simulink model "sim_model"  (R2015b)
settings: Solver=FixedStepDiscrete  SolverMode=SingleTasking  StartTime=0.0  StopTime=sim_len  FixedStep=1  RelTol=1e-3
values from neighbouring files (symbols this model uses):
  N_sub = 16    [channelizer_params.m]    (also in channelizer_params_256.m = 256; channelizer_params_512.m = 512)
undefined symbols (not defined in the file or in its folder): modulator_reg_1_address, modulator_reg_1_default, modulator_reg_1_num_bits
libraries: xbsIndex_r4 x150
(part 1 of 2)
settings Model: Creator=randy  LastModifiedBy=randy

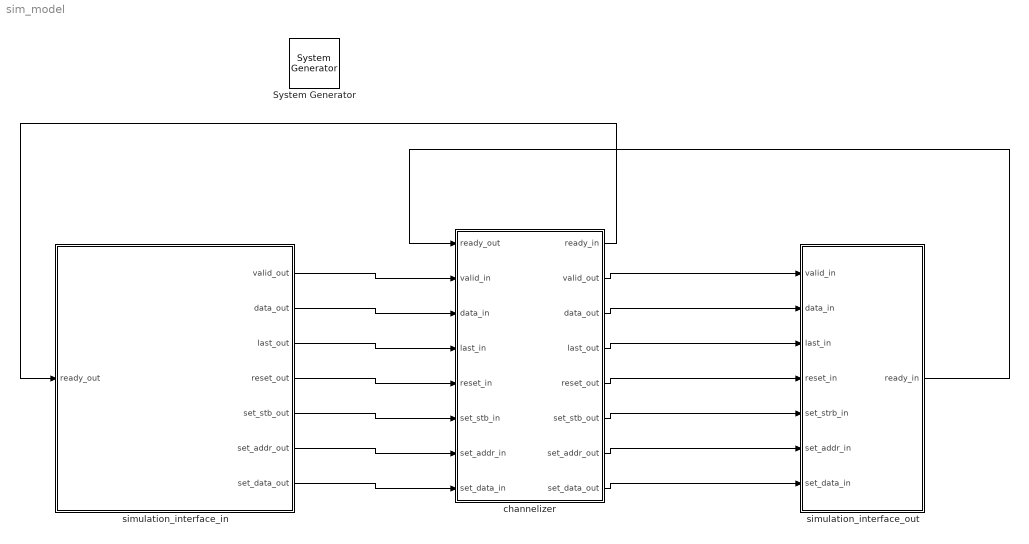
== system sim_model ==
  " System Generator" : xbsIndex_r4/ System Generator  Tag=genX  xilinxfamily=kintex7  part=xc7k325t  speed=-3  package=fbg676  synthesis_tool=Vivado  clock_wrapper=Clock Enables  directory=./netlist  proj_type=Vivado  Synth_file=Vivado Synthesis Defaults  Impl_file=Vivado Implementation Defaults  testbench=off  simulink_period=1  sysclk_period=10  dcm_input_clock_period=10  incr_netlist=off  trim_vbits=Everywhere in SubSystem  dbl_ovrd=According to Block Masks  core_generation=According to Block Masks  run_coregen=off  deprecated_control=off  eval_field=0  block_type=sysgen
  channelizer : Subsystem
  simulation_interface_in : Subsystem
  simulation_interface_out : Subsystem
  wires:
  channelizer/1(ready_in) -> simulation_interface_in/1(ready_out)
  channelizer/2(valid_out) -> simulation_interface_out/1(valid_in)
  channelizer/3(data_out) -> simulation_interface_out/2(data_in)
  channelizer/4(last_out) -> simulation_interface_out/3(last_in)
  simulation_interface_out/1(ready_in) -> channelizer/1(ready_out)
  channelizer/5(reset_out) -> simulation_interface_out/4(reset_in)
  channelizer/6(set_stb_out) -> simulation_interface_out/5(set_strb_in)
  channelizer/7(set_addr_out) -> simulation_interface_out/6(set_addr_in)
  channelizer/8(set_data_out) -> simulation_interface_out/7(set_data_in)
  simulation_interface_in/1(valid_out) -> channelizer/2(valid_in)
  simulation_interface_in/2(data_out) -> channelizer/3(data_in)
  simulation_interface_in/3(last_out) -> channelizer/4(last_in)
  simulation_interface_in/4(reset_out) -> channelizer/5(reset_in)
  simulation_interface_in/5(set_stb_out) -> channelizer/6(set_stb_in)
  simulation_interface_in/6(set_addr_out) -> channelizer/7(set_addr_in)
  simulation_interface_in/7(set_data_out) -> channelizer/8(set_data_in)

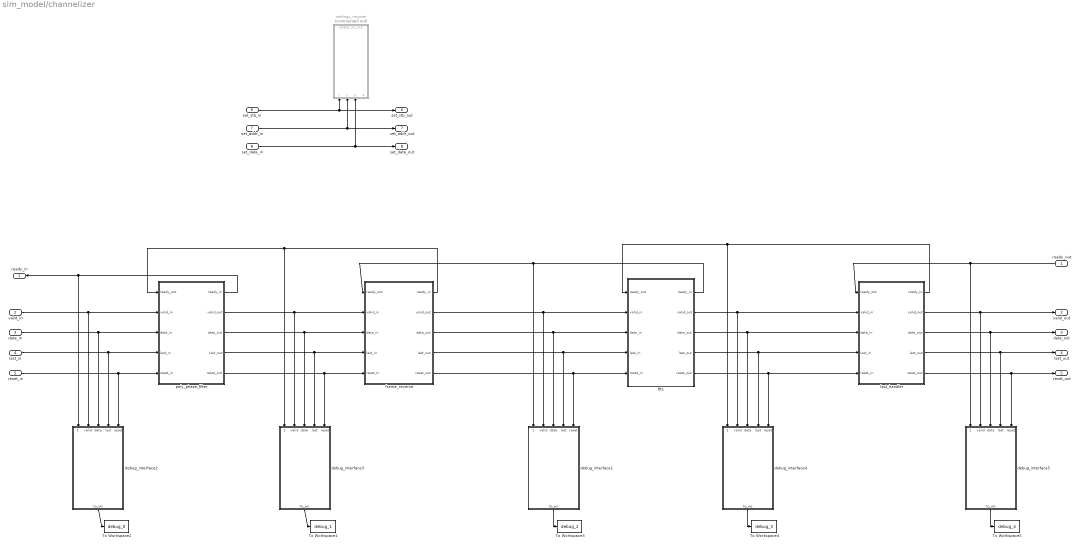
== system sim_model/channelizer ==
  ready_out : Inport
  valid_in : Inport  Port=2
  data_in : Inport  Port=3
  last_in : Inport  Port=4
  reset_in : Inport  Port=5
  set_stb_in : Inport  Port=6
  set_addr_in : Inport  Port=7
  set_data_in : Inport  Port=8
  To Workspace1 : ToWorkspace  VariableName=debug_1  SaveFormat=Timeseries  SampleTime=-1
  To Workspace2 : ToWorkspace  VariableName=debug_0  SaveFormat=Timeseries  SampleTime=-1
  To Workspace3 : ToWorkspace  VariableName=debug_2  SaveFormat=Timeseries  SampleTime=-1
  To Workspace4 : ToWorkspace  VariableName=debug_3  SaveFormat=Timeseries  SampleTime=-1
  To Workspace5 : ToWorkspace  VariableName=debug_4  SaveFormat=Timeseries  SampleTime=-1
  debug_interface1 : Subsystem
  debug_interface2 : Subsystem
  debug_interface3 : Subsystem
  debug_interface4 : Subsystem
  debug_interface5 : Subsystem
  fft1 : Subsystem
  frame_reverse : Subsystem
  last_handler : Subsystem
  poly_phase_filter : Subsystem
  settings_register : Subsystem  Commented=on
  ready_in : Outport
  valid_out : Outport  Port=2
  data_out : Outport  Port=3
  last_out : Outport  Port=4
  reset_out : Outport  Port=5
  set_stb_out : Outport  Port=6
  set_addr_out : Outport  Port=7
  set_data_out : Outport  Port=8
  wires:
  set_stb_in/1 -> settings_register/1(set_stb), set_stb_out/1
  set_addr_in/1 -> settings_register/2(set_addr), set_addr_out/1
  set_data_in/1 -> settings_register/3(set_data), set_data_out/1
  debug_interface2/1(to_ws) -> To Workspace2/1
  debug_interface3/1(to_ws) -> To Workspace1/1
  debug_interface1/1(to_ws) -> To Workspace3/1
  debug_interface4/1(to_ws) -> To Workspace4/1
  poly_phase_filter/1(ready_in) -> debug_interface2/1(ready), ready_in/1
  data_in/1 -> poly_phase_filter/3(data_in), debug_interface2/3(data)
  valid_in/1 -> poly_phase_filter/2(valid_in), debug_interface2/2(valid)
  last_in/1 -> poly_phase_filter/4(last_in), debug_interface2/4(last)
  reset_in/1 -> poly_phase_filter/5(reset_in), debug_interface2/5(reset)
  poly_phase_filter/2(valid_out) -> frame_reverse/2(valid_in), debug_interface3/2(valid)
  poly_phase_filter/3(data_out) -> frame_reverse/3(data_in), debug_interface3/3(data)
  poly_phase_filter/4(last_out) -> frame_reverse/4(last_in), debug_interface3/4(last)
  poly_phase_filter/5(reset_out) -> debug_interface3/5(reset), frame_reverse/5(reset_in)
  frame_reverse/2(valid_out) -> fft1/2(valid_in), debug_interface1/2(valid)
  frame_reverse/4(last_out) -> fft1/4(last_in), debug_interface1/4(last)
  frame_reverse/5(reset_out) -> fft1/5(reset_in), debug_interface1/5(reset)
  fft1/1(ready_in) -> frame_reverse/1(ready_out), debug_interface1/1(ready)
  frame_reverse/3(data_out) -> fft1/3(data_in), debug_interface1/3(data)
  frame_reverse/1(ready_in) -> poly_phase_filter/1(ready_out), debug_interface3/1(ready)
  last_handler/5(reset_out) -> reset_out/1, debug_interface5/5(reset)
  last_handler/4(last_out) -> last_out/1, debug_interface5/4(last)
  last_handler/3(data_out) -> data_out/1, debug_interface5/3(data)
  fft1/2(valid_out) -> debug_interface4/2(valid), last_handler/2(valid_in)
  fft1/3(data_out) -> debug_interface4/3(data), last_handler/3(data_in)
  fft1/4(last_out) -> debug_interface4/4(last), last_handler/4(last_in)
  fft1/5(reset_out) -> debug_interface4/5(reset), last_handler/5(reset_in)
  last_handler/2(valid_out) -> debug_interface5/2(valid), valid_out/1
  ready_out/1 -> debug_interface5/1(ready), last_handler/1(ready_out)
  last_handler/1(ready_in) -> debug_interface4/1(ready), fft1/1(ready_out)
  debug_interface5/1(to_ws) -> To Workspace5/1

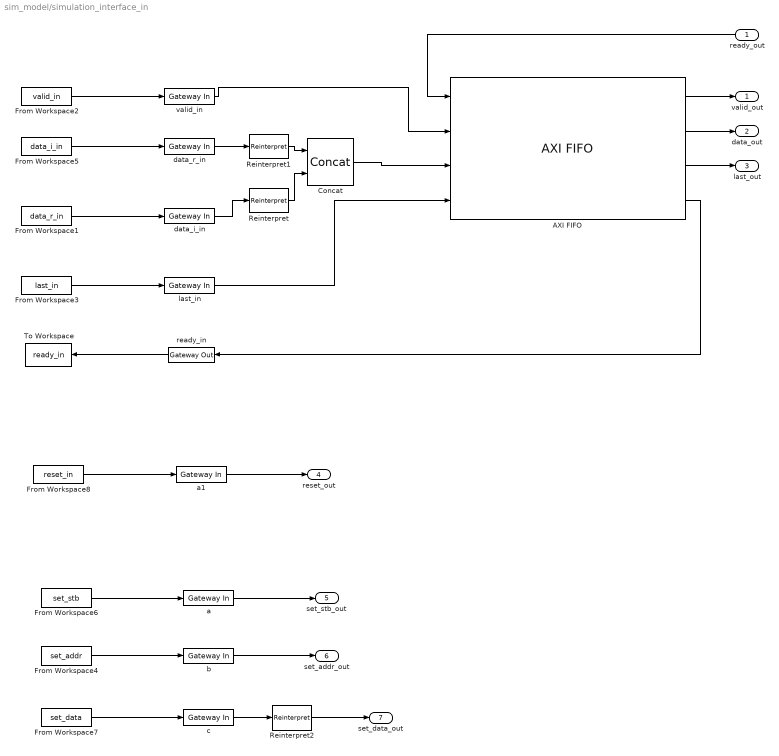
== system sim_model/simulation_interface_in ==
  ready_out : Inport
  AXI FIFO : xbsIndex_r4/AXI FIFO  input_depth_axis=16K  actual_fifo_depth_label=16386  enable_tdata=on  enable_tdest=off  enable_tstrb=off  enable_tready=on  enable_tid=off  enable_tuser=off  enable_tkeep=off  enable_tlast=on  has_aresetn=off  enable_data_counts_axis=off  fifo_implementation_type_axis=Common Clock Block RAM  trim_axipin_name=on  programmable_full_type_axis=Full  full_threshold_assert_value_axis=0  programmable_empty_type_axis=Empty  empty_threshold_assert_value_axis=1022  underflow_flag_axi=0  underflow_sense_axi=Active High  overflow_flag_axi=0  overflow_sense_axi=Active High  block_type=axi_fifo
  Concat : xbsIndex_r4/Concat  num_inputs=2  dbl_ovrd=off  block_type=concat
  From Workspace1 : FromWorkspace  VariableName=data_r_in  SampleTime=0
  From Workspace2 : FromWorkspace  VariableName=valid_in  SampleTime=0
  From Workspace3 : FromWorkspace  VariableName=last_in  SampleTime=0
  From Workspace4 : FromWorkspace  VariableName=set_addr  SampleTime=0
  From Workspace5 : FromWorkspace  VariableName=data_i_in  SampleTime=0
  From Workspace6 : FromWorkspace  VariableName=set_stb  SampleTime=0
  From Workspace7 : FromWorkspace  VariableName=set_data  SampleTime=0
  From Workspace8 : FromWorkspace  VariableName=reset_in  SampleTime=0
  Reinterpret : xbsIndex_r4/Reinterpret  force_arith_type=on  arith_type=Unsigned  force_bin_pt=on  bin_pt=0  block_type=reinterpret
  Reinterpret1 : xbsIndex_r4/Reinterpret  force_arith_type=on  arith_type=Unsigned  force_bin_pt=on  bin_pt=0  block_type=reinterpret
  Reinterpret2 : xbsIndex_r4/Reinterpret  force_arith_type=on  arith_type=Unsigned  force_bin_pt=on  bin_pt=0  block_type=reinterpret
  To Workspace : ToWorkspace  VariableName=ready_in  SaveFormat=Timeseries  SampleTime=-1
  a : xbsIndex_r4/Gateway In  gui_display_data_type=Boolean  arith_type=Boolean  n_bits=16  bin_pt=14  preci_type=Single  exp_width=8  frac_width=24  rows=1  columns=1  quantization="Round  (unbiased: +/- Inf)"  overflow=Saturate  period=1  UseAsADC=off  ADCChannel='1'  interface=None  automatic_assignment=on  address_offset=hex2dec('00')  intf_name=''  intf_description=''  timing_constraint=None  locs_specified=off  LOCs={}  io_standard={}  inherit_from_input=off  hdl_port=on  dbl_ovrd=off  block_type=gatewayin
  a1 : xbsIndex_r4/Gateway In  gui_display_data_type=Boolean  arith_type=Boolean  n_bits=16  bin_pt=14  preci_type=Single  exp_width=8  frac_width=24  rows=1  columns=1  quantization="Round  (unbiased: +/- Inf)"  overflow=Saturate  period=1  UseAsADC=off  ADCChannel='1'  interface=None  automatic_assignment=on  address_offset=hex2dec('00')  intf_name=''  intf_description=''  timing_constraint=None  locs_specified=off  LOCs={}  io_standard={}  inherit_from_input=off  hdl_port=on  dbl_ovrd=off  block_type=gatewayin
  b : xbsIndex_r4/Gateway In  gui_display_data_type=Fixed-point  arith_type=Unsigned  n_bits=8  bin_pt=0  preci_type=Single  exp_width=8  frac_width=24  rows=1  columns=1  quantization="Round  (unbiased: +/- Inf)"  overflow=Saturate  period=1  UseAsADC=off  ADCChannel='1'  interface=None  automatic_assignment=on  address_offset=hex2dec('00')  intf_name=''  intf_description=''  timing_constraint=None  locs_specified=off  LOCs={}  io_standard={}  inherit_from_input=off  hdl_port=on  dbl_ovrd=off  block_type=gatewayin
  c : xbsIndex_r4/Gateway In  gui_display_data_type=Fixed-point  arith_type=Unsigned  n_bits=32  bin_pt=0  preci_type=Single  exp_width=8  frac_width=24  rows=1  columns=1  quantization="Round  (unbiased: +/- Inf)"  overflow=Saturate  period=1  UseAsADC=off  ADCChannel='1'  interface=None  automatic_assignment=on  address_offset=hex2dec('00')  intf_name=''  intf_description=''  timing_constraint=None  locs_specified=off  LOCs={}  io_standard={}  inherit_from_input=off  hdl_port=on  dbl_ovrd=off  block_type=gatewayin
  data_i_in : xbsIndex_r4/Gateway In  gui_display_data_type=Fixed-point  arith_type="Signed  (2's comp)"  n_bits=16  bin_pt=15  preci_type=Single  exp_width=8  frac_width=24  rows=1  columns=1  quantization="Round  (unbiased: +/- Inf)"  overflow=Saturate  period=1  UseAsADC=off  ADCChannel='1'  interface=None  automatic_assignment=on  address_offset=hex2dec('00')  intf_name=''  intf_description=''  timing_constraint=None  locs_specified=off  LOCs={}  io_standard={}  inherit_from_input=off  hdl_port=on  dbl_ovrd=off  block_type=gatewayin
  data_r_in : xbsIndex_r4/Gateway In  gui_display_data_type=Fixed-point  arith_type="Signed  (2's comp)"  n_bits=16  bin_pt=15  preci_type=Single  exp_width=8  frac_width=24  rows=1  columns=1  quantization="Round  (unbiased: +/- Inf)"  overflow=Saturate  period=1  UseAsADC=off  ADCChannel='1'  interface=None  automatic_assignment=on  address_offset=hex2dec('00')  intf_name=''  intf_description=''  timing_constraint=None  locs_specified=off  LOCs={}  io_standard={}  inherit_from_input=off  hdl_port=on  dbl_ovrd=off  block_type=gatewayin
  last_in : xbsIndex_r4/Gateway In  gui_display_data_type=Boolean  arith_type=Boolean  n_bits=16  bin_pt=14  preci_type=Single  exp_width=8  frac_width=24  rows=1  columns=1  quantization="Round  (unbiased: +/- Inf)"  overflow=Saturate  period=1  UseAsADC=off  ADCChannel='1'  interface=None  automatic_assignment=on  address_offset=hex2dec('00')  intf_name=''  intf_description=''  timing_constraint=None  locs_specified=off  LOCs={}  io_standard={}  inherit_from_input=off  hdl_port=on  dbl_ovrd=off  block_type=gatewayin
  ready_in : xbsIndex_r4/Gateway Out  inherit_from_input=off  hdl_port=on  rows=1  columns=1  UseAsDAC=off  DACChannel='1'  interface=None  automatic_assignment=on  address_offset=hex2dec('00')  intf_name=''  intf_description=''  timing_constraint=None  locs_specified=off  LOCs={}  io_standard={}  block_type=gatewayout
  valid_in : xbsIndex_r4/Gateway In  gui_display_data_type=Boolean  arith_type=Boolean  n_bits=16  bin_pt=14  preci_type=Single  exp_width=8  frac_width=24  rows=1  columns=1  quantization="Round  (unbiased: +/- Inf)"  overflow=Saturate  period=1  UseAsADC=off  ADCChannel='1'  interface=None  automatic_assignment=on  address_offset=hex2dec('00')  intf_name=''  intf_description=''  timing_constraint=None  locs_specified=off  LOCs={}  io_standard={}  inherit_from_input=off  hdl_port=on  dbl_ovrd=off  block_type=gatewayin
  valid_out : Outport
  data_out : Outport  Port=2
  last_out : Outport  Port=3
  reset_out : Outport  Port=4
  set_stb_out : Outport  Port=5
  set_addr_out : Outport  Port=6
  set_data_out : Outport  Port=7
  wires:
  ready_out/1 -> AXI FIFO/1
  AXI FIFO/2 -> data_out/1
  AXI FIFO/3 -> last_out/1
  AXI FIFO/1 -> valid_out/1
  From Workspace2/1 -> valid_in/1
  From Workspace3/1 -> last_in/1
  ready_in/1 -> To Workspace/1
  AXI FIFO/4 -> ready_in/1
  last_in/1 -> AXI FIFO/4
  valid_in/1 -> AXI FIFO/2
  data_i_in/1 -> Reinterpret/1
  data_r_in/1 -> Reinterpret1/1
  From Workspace5/1 -> data_r_in/1
  Concat/1 -> AXI FIFO/3
  From Workspace1/1 -> data_i_in/1
  From Workspace6/1 -> a/1
  From Workspace4/1 -> b/1
  From Workspace7/1 -> c/1
  c/1 -> Reinterpret2/1
  a/1 -> set_stb_out/1
  b/1 -> set_addr_out/1
  Reinterpret2/1 -> set_data_out/1
  From Workspace8/1 -> a1/1
  a1/1 -> reset_out/1
  Reinterpret1/1 -> Concat/1
  Reinterpret/1 -> Concat/2

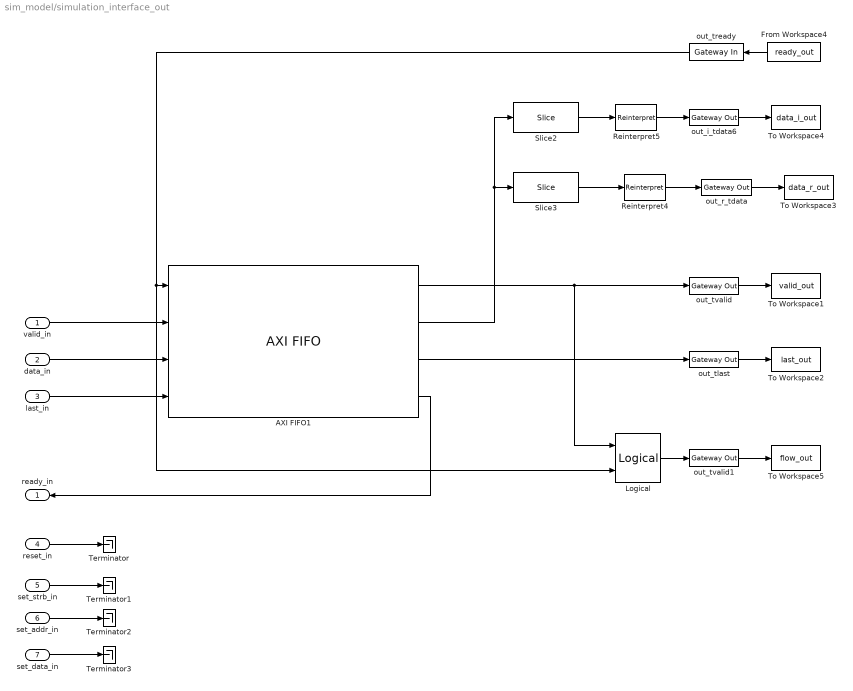
== system sim_model/simulation_interface_out ==
  valid_in : Inport
  data_in : Inport  Port=2
  last_in : Inport  Port=3
  reset_in : Inport  Port=4
  set_strb_in : Inport  Port=5
  set_addr_in : Inport  Port=6
  set_data_in : Inport  Port=7
  AXI FIFO1 : xbsIndex_r4/AXI FIFO  input_depth_axis=32  actual_fifo_depth_label=34  enable_tdata=on  enable_tdest=off  enable_tstrb=off  enable_tready=on  enable_tid=off  enable_tuser=off  enable_tkeep=off  enable_tlast=on  has_aresetn=off  enable_data_counts_axis=off  fifo_implementation_type_axis=Common Clock Block RAM  trim_axipin_name=on  programmable_full_type_axis=Full  full_threshold_assert_value_axis=0  programmable_empty_type_axis=Empty  empty_threshold_assert_value_axis=1022  underflow_flag_axi=0  underflow_sense_axi=Active High  overflow_flag_axi=0  overflow_sense_axi=Active High  block_type=axi_fifo
  From Workspace4 : FromWorkspace  VariableName=ready_out  SampleTime=0
  Logical : xbsIndex_r4/Logical  logical_function=AND  inputs=2  en=off  latency=0  precision=Full  arith_type=Unsigned  n_bits=16  bin_pt=0  align_bp=on  dbl_ovrd=off  block_type=logical
  Reinterpret4 : xbsIndex_r4/Reinterpret  force_arith_type=on  arith_type="Signed  (2's comp)"  force_bin_pt=on  bin_pt=14  block_type=reinterpret
  Reinterpret5 : xbsIndex_r4/Reinterpret  force_arith_type=on  arith_type="Signed  (2's comp)"  force_bin_pt=on  bin_pt=14  block_type=reinterpret
  Slice2 : xbsIndex_r4/Slice  nbits=16  boolean_output=off  mode=Two Bit Locations  bit1=15  base1=LSB of Input  bit0=0  base0=LSB of Input  dbl_ovrd=off  block_type=slice
  Slice3 : xbsIndex_r4/Slice  nbits=16  boolean_output=off  mode=Two Bit Locations  bit1=31  base1=LSB of Input  bit0=16  base0=LSB of Input  dbl_ovrd=off  block_type=slice
  Terminator{,1..3} (4 alike) : Terminator
  To Workspace1 : ToWorkspace  VariableName=valid_out  SaveFormat=Timeseries  SampleTime=-1
  To Workspace2 : ToWorkspace  VariableName=last_out  SaveFormat=Timeseries  SampleTime=-1
  To Workspace3 : ToWorkspace  VariableName=data_r_out  SaveFormat=Timeseries  SampleTime=-1
  To Workspace4 : ToWorkspace  VariableName=data_i_out  SaveFormat=Timeseries  SampleTime=-1
  To Workspace5 : ToWorkspace  VariableName=flow_out  SaveFormat=Timeseries  SampleTime=-1
  out_i_tdata6 : xbsIndex_r4/Gateway Out  inherit_from_input=off  hdl_port=on  rows=1  columns=1  UseAsDAC=off  DACChannel='1'  interface=None  automatic_assignment=on  address_offset=hex2dec('00')  intf_name=''  intf_description=''  timing_constraint=None  locs_specified=off  LOCs={}  io_standard={}  block_type=gatewayout
  out_r_tdata : xbsIndex_r4/Gateway Out  inherit_from_input=off  hdl_port=on  rows=1  columns=1  UseAsDAC=off  DACChannel='1'  interface=None  automatic_assignment=on  address_offset=hex2dec('00')  intf_name=''  intf_description=''  timing_constraint=None  locs_specified=off  LOCs={}  io_standard={}  block_type=gatewayout
  out_tlast : xbsIndex_r4/Gateway Out  inherit_from_input=off  hdl_port=on  rows=1  columns=1  UseAsDAC=off  DACChannel='1'  interface=None  automatic_assignment=on  address_offset=hex2dec('00')  intf_name=''  intf_description=''  timing_constraint=None  locs_specified=off  LOCs={}  io_standard={}  block_type=gatewayout
  out_tready : xbsIndex_r4/Gateway In  gui_display_data_type=Boolean  arith_type=Boolean  n_bits=16  bin_pt=14  preci_type=Single  exp_width=8  frac_width=24  rows=1  columns=1  quantization="Round  (unbiased: +/- Inf)"  overflow=Saturate  period=1  UseAsADC=off  ADCChannel='1'  interface=None  automatic_assignment=on  address_offset=hex2dec('00')  intf_name=''  intf_description=''  timing_constraint=None  locs_specified=off  LOCs={}  io_standard={}  inherit_from_input=off  hdl_port=on  dbl_ovrd=off  block_type=gatewayin
  out_tvalid : xbsIndex_r4/Gateway Out  inherit_from_input=off  hdl_port=on  rows=1  columns=1  UseAsDAC=off  DACChannel='1'  interface=None  automatic_assignment=on  address_offset=hex2dec('00')  intf_name=''  intf_description=''  timing_constraint=None  locs_specified=off  LOCs={}  io_standard={}  block_type=gatewayout
  out_tvalid1 : xbsIndex_r4/Gateway Out  inherit_from_input=off  hdl_port=on  rows=1  columns=1  UseAsDAC=off  DACChannel='1'  interface=None  automatic_assignment=on  address_offset=hex2dec('00')  intf_name=''  intf_description=''  timing_constraint=None  locs_specified=off  LOCs={}  io_standard={}  block_type=gatewayout
  ready_in : Outport
  wires:
  AXI FIFO1/4 -> ready_in/1
  valid_in/1 -> AXI FIFO1/2
  data_in/1 -> AXI FIFO1/3
  last_in/1 -> AXI FIFO1/4
  AXI FIFO1/1 -> Logical/1, out_tvalid/1
  AXI FIFO1/3 -> out_tlast/1
  out_tvalid/1 -> To Workspace1/1
  From Workspace4/1 -> out_tready/1
  out_tlast/1 -> To Workspace2/1
  Reinterpret4/1 -> out_r_tdata/1
  Reinterpret5/1 -> out_i_tdata6/1
  AXI FIFO1/2 -> Slice2/1, Slice3/1
  out_r_tdata/1 -> To Workspace3/1
  out_i_tdata6/1 -> To Workspace4/1
  out_tready/1 -> Logical/2, AXI FIFO1/1
  out_tvalid1/1 -> To Workspace5/1
  Logical/1 -> out_tvalid1/1
  Slice2/1 -> Reinterpret5/1
  Slice3/1 -> Reinterpret4/1
  reset_in/1 -> Terminator/1
  set_strb_in/1 -> Terminator1/1
  set_addr_in/1 -> Terminator2/1
  set_data_in/1 -> Terminator3/1

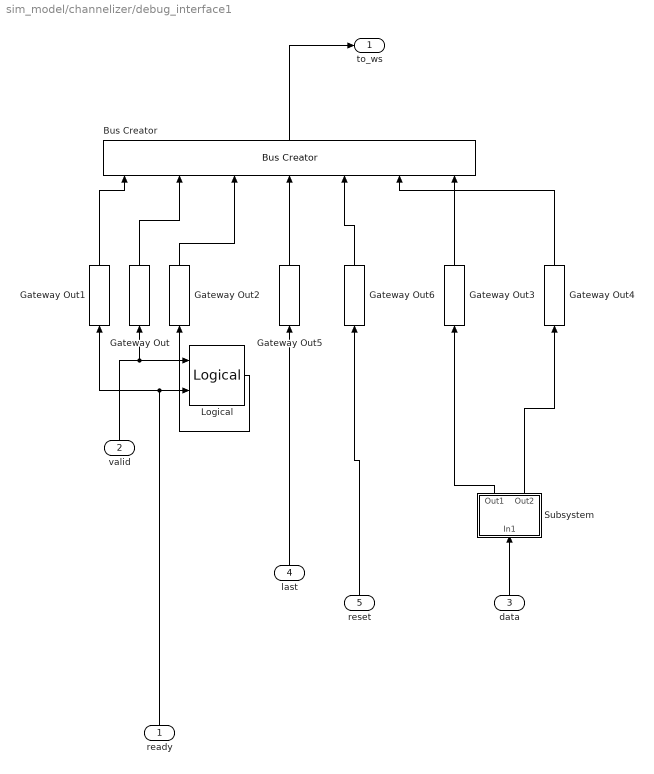
== system sim_model/channelizer/debug_interface1 ==
  ready : Inport
  valid : Inport  Port=2
  data : Inport  Port=3
  last : Inport  Port=4
  reset : Inport  Port=5
  Bus Creator : BusCreator  Inputs=7
  Gateway Out{,1..6} (7 alike) : xbsIndex_r4/Gateway Out  inherit_from_input=off  hdl_port=off  rows=1  columns=1  UseAsDAC=off  DACChannel='1'  interface=None  automatic_assignment=on  address_offset=hex2dec('00')  intf_name=''  intf_description=''  timing_constraint=None  locs_specified=off  LOCs={}  io_standard={}  block_type=gatewayout
  Logical : xbsIndex_r4/Logical  logical_function=AND  inputs=2  en=off  latency=0  precision=Full  arith_type=Unsigned  n_bits=16  bin_pt=0  align_bp=on  dbl_ovrd=off  block_type=logical
  Subsystem : Subsystem
  to_ws : Outport
  wires:
  ready/1 -> Logical/2, Gateway Out1/1
  Gateway Out3/1 -> Bus Creator/7
  Gateway Out2/1 -> Bus Creator/3
  Logical/1 -> Gateway Out2/1
  Gateway Out4/1 -> Bus Creator/6
  valid/1 -> Logical/1, Gateway Out/1
  Gateway Out1/1 -> Bus Creator/1
  Gateway Out/1 -> Bus Creator/2
  Gateway Out6/1 -> Bus Creator/5
  reset/1 -> Gateway Out6/1
  Bus Creator/1 -> to_ws/1
  Subsystem/1(Out1) -> Gateway Out3/1
  Subsystem/2(Out2) -> Gateway Out4/1
  data/1 -> Subsystem/1(In1)
  Gateway Out5/1 -> Bus Creator/4
  last/1 -> Gateway Out5/1

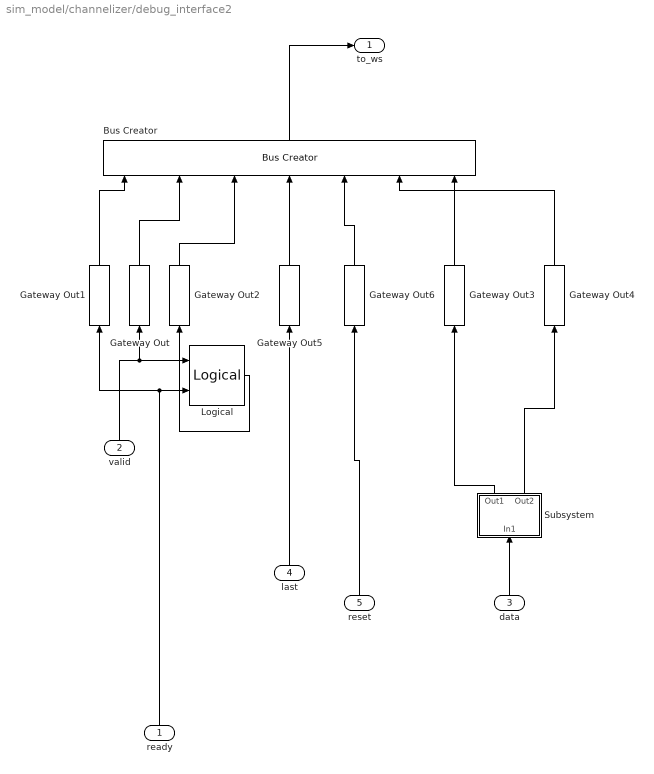
== system sim_model/channelizer/debug_interface2 ==
  ready : Inport
  valid : Inport  Port=2
  data : Inport  Port=3
  last : Inport  Port=4
  reset : Inport  Port=5
  Bus Creator : BusCreator  Inputs=7
  Gateway Out{,1..6} (7 alike) : xbsIndex_r4/Gateway Out  inherit_from_input=off  hdl_port=off  rows=1  columns=1  UseAsDAC=off  DACChannel='1'  interface=None  automatic_assignment=on  address_offset=hex2dec('00')  intf_name=''  intf_description=''  timing_constraint=None  locs_specified=off  LOCs={}  io_standard={}  block_type=gatewayout
  Logical : xbsIndex_r4/Logical  logical_function=AND  inputs=2  en=off  latency=0  precision=Full  arith_type=Unsigned  n_bits=16  bin_pt=0  align_bp=on  dbl_ovrd=off  block_type=logical
  Subsystem : Subsystem
  to_ws : Outport
  wires:
  ready/1 -> Logical/2, Gateway Out1/1
  Gateway Out3/1 -> Bus Creator/7
  Gateway Out2/1 -> Bus Creator/3
  Logical/1 -> Gateway Out2/1
  Gateway Out4/1 -> Bus Creator/6
  valid/1 -> Logical/1, Gateway Out/1
  Gateway Out1/1 -> Bus Creator/1
  Gateway Out/1 -> Bus Creator/2
  Gateway Out6/1 -> Bus Creator/5
  reset/1 -> Gateway Out6/1
  Bus Creator/1 -> to_ws/1
  Subsystem/1(Out1) -> Gateway Out3/1
  Subsystem/2(Out2) -> Gateway Out4/1
  data/1 -> Subsystem/1(In1)
  Gateway Out5/1 -> Bus Creator/4
  last/1 -> Gateway Out5/1

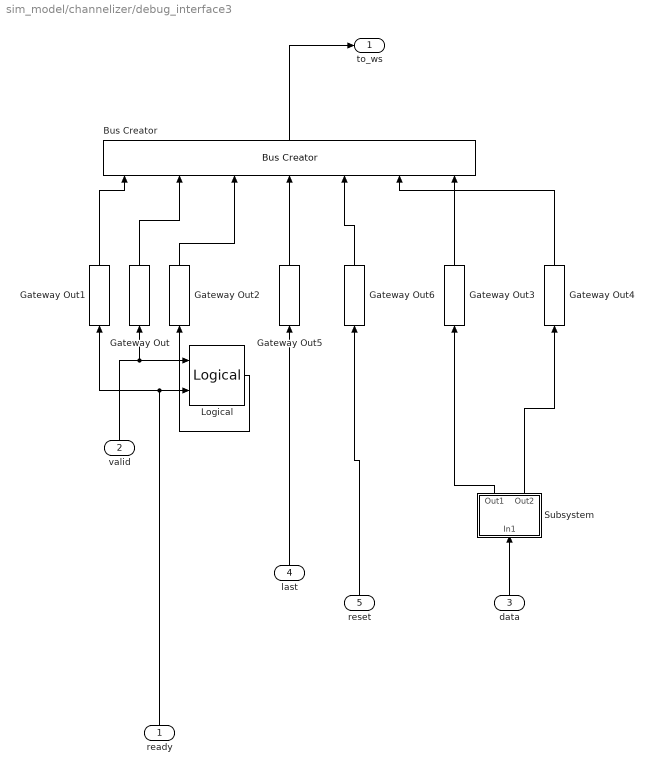
== system sim_model/channelizer/debug_interface3 ==
  ready : Inport
  valid : Inport  Port=2
  data : Inport  Port=3
  last : Inport  Port=4
  reset : Inport  Port=5
  Bus Creator : BusCreator  Inputs=7
  Gateway Out{,1..6} (7 alike) : xbsIndex_r4/Gateway Out  inherit_from_input=off  hdl_port=off  rows=1  columns=1  UseAsDAC=off  DACChannel='1'  interface=None  automatic_assignment=on  address_offset=hex2dec('00')  intf_name=''  intf_description=''  timing_constraint=None  locs_specified=off  LOCs={}  io_standard={}  block_type=gatewayout
  Logical : xbsIndex_r4/Logical  logical_function=AND  inputs=2  en=off  latency=0  precision=Full  arith_type=Unsigned  n_bits=16  bin_pt=0  align_bp=on  dbl_ovrd=off  block_type=logical
  Subsystem : Subsystem
  to_ws : Outport
  wires:
  last/1 -> Gateway Out5/1
  Gateway Out5/1 -> Bus Creator/4
  data/1 -> Subsystem/1(In1)
  Subsystem/2(Out2) -> Gateway Out4/1
  Subsystem/1(Out1) -> Gateway Out3/1
  Bus Creator/1 -> to_ws/1
  reset/1 -> Gateway Out6/1
  Gateway Out6/1 -> Bus Creator/5
  Gateway Out/1 -> Bus Creator/2
  Gateway Out1/1 -> Bus Creator/1
  valid/1 -> Gateway Out/1, Logical/1
  Gateway Out4/1 -> Bus Creator/6
  Logical/1 -> Gateway Out2/1
  Gateway Out2/1 -> Bus Creator/3
  Gateway Out3/1 -> Bus Creator/7
  ready/1 -> Gateway Out1/1, Logical/2

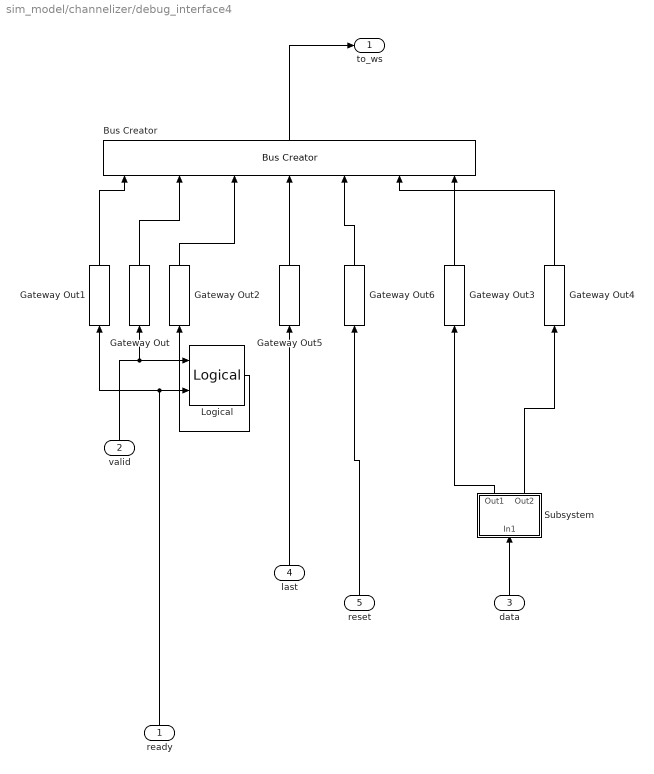
== system sim_model/channelizer/debug_interface4 ==
  ready : Inport
  valid : Inport  Port=2
  data : Inport  Port=3
  last : Inport  Port=4
  reset : Inport  Port=5
  Bus Creator : BusCreator  Inputs=7
  Gateway Out{,1..6} (7 alike) : xbsIndex_r4/Gateway Out  inherit_from_input=off  hdl_port=off  rows=1  columns=1  UseAsDAC=off  DACChannel='1'  interface=None  automatic_assignment=on  address_offset=hex2dec('00')  intf_name=''  intf_description=''  timing_constraint=None  locs_specified=off  LOCs={}  io_standard={}  block_type=gatewayout
  Logical : xbsIndex_r4/Logical  logical_function=AND  inputs=2  en=off  latency=0  precision=Full  arith_type=Unsigned  n_bits=16  bin_pt=0  align_bp=on  dbl_ovrd=off  block_type=logical
  Subsystem : Subsystem
  to_ws : Outport
  wires:
  ready/1 -> Logical/2, Gateway Out1/1
  Gateway Out3/1 -> Bus Creator/7
  Gateway Out2/1 -> Bus Creator/3
  Logical/1 -> Gateway Out2/1
  Gateway Out4/1 -> Bus Creator/6
  valid/1 -> Logical/1, Gateway Out/1
  Gateway Out1/1 -> Bus Creator/1
  Gateway Out/1 -> Bus Creator/2
  Gateway Out6/1 -> Bus Creator/5
  reset/1 -> Gateway Out6/1
  Bus Creator/1 -> to_ws/1
  Subsystem/1(Out1) -> Gateway Out3/1
  Subsystem/2(Out2) -> Gateway Out4/1
  data/1 -> Subsystem/1(In1)
  Gateway Out5/1 -> Bus Creator/4
  last/1 -> Gateway Out5/1

== system sim_model/channelizer/debug_interface5 ==
  ready : Inport
  valid : Inport  Port=2
  data : Inport  Port=3
  last : Inport  Port=4
  reset : Inport  Port=5
  Bus Creator : BusCreator  Inputs=7
  Gateway Out{,1..6} (7 alike) : xbsIndex_r4/Gateway Out  inherit_from_input=off  hdl_port=off  rows=1  columns=1  UseAsDAC=off  DACChannel='1'  interface=None  automatic_assignment=on  address_offset=hex2dec('00')  intf_name=''  intf_description=''  timing_constraint=None  locs_specified=off  LOCs={}  io_standard={}  block_type=gatewayout
  Logical : xbsIndex_r4/Logical  logical_function=AND  inputs=2  en=off  latency=0  precision=Full  arith_type=Unsigned  n_bits=16  bin_pt=0  align_bp=on  dbl_ovrd=off  block_type=logical
  Subsystem : Subsystem
  to_ws : Outport
  wires:
  ready/1 -> Logical/2, Gateway Out1/1
  Gateway Out3/1 -> Bus Creator/7
  Gateway Out2/1 -> Bus Creator/3
  Logical/1 -> Gateway Out2/1
  Gateway Out4/1 -> Bus Creator/6
  valid/1 -> Logical/1, Gateway Out/1
  Gateway Out1/1 -> Bus Creator/1
  Gateway Out/1 -> Bus Creator/2
  Gateway Out6/1 -> Bus Creator/5
  reset/1 -> Gateway Out6/1
  Bus Creator/1 -> to_ws/1
  Subsystem/1(Out1) -> Gateway Out3/1
  Subsystem/2(Out2) -> Gateway Out4/1
  data/1 -> Subsystem/1(In1)
  Gateway Out5/1 -> Bus Creator/4
  last/1 -> Gateway Out5/1

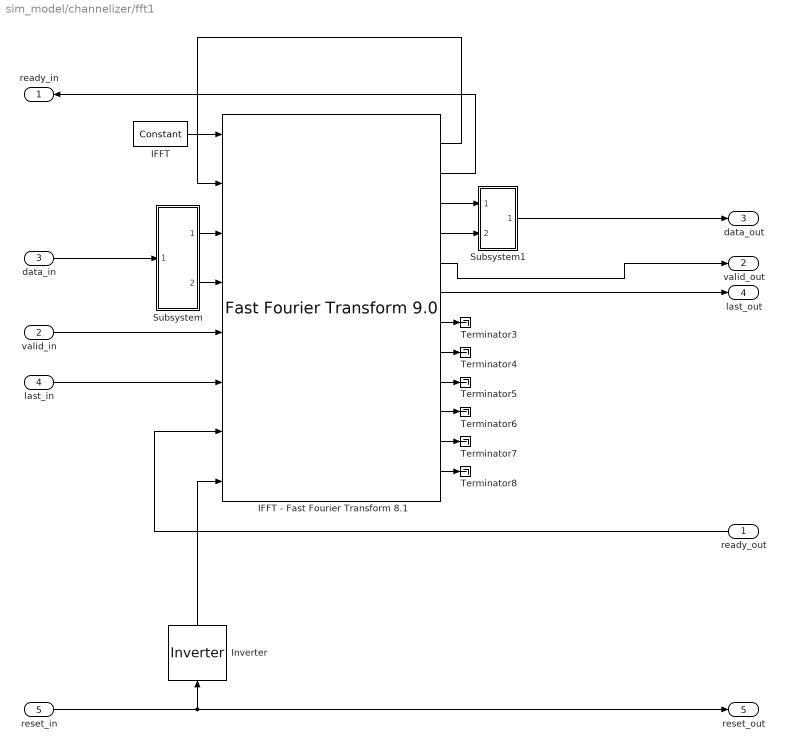
== system sim_model/channelizer/fft1 ==
  ready_out : Inport
  valid_in : Inport  Port=2
  data_in : Inport  Port=3
  last_in : Inport  Port=4
  reset_in : Inport  Port=5
  IFFT : xbsIndex_r4/Constant  const=1  gui_display_data_type=Fixed-point  arith_type=Unsigned  n_bits=1  bin_pt=0  preci_type=Single  exp_width=8  frac_width=24  explicit_period=off  period=1  equ=P=C  opselect=C  inp2=PCIN>>17  opr=+  inp1=P  carry=CIN  dbl_ovrd=off  block_type=constant
  IFFT - Fast Fourier Transform 8.1 : xbsIndex_r4/Fast Fourier Transform 9.0   transform_length=16  target_clock_frequency=250  target_data_throughput=50  implementation_options=pipelined_streaming_io  run_time_configurable_transform_length=off  phase_factor_width=17  scaling_options=unscaled  rounding_modes=convergent_rounding  aclken=off  aresetn=on  cyclic_prefix_insertion=off  output_ordering=natural_order  throttle_scheme=nonrealtime  xk_index=off  ovflo=off  trim_axipin_name=on  memory_options_data=block_ram  memory_options_phase_factors=block_ram  number_of_stages_using_block_ram_for_data_and_phase_factors=0  memory_options_reorder=block_ram  memory_options_hybrid=off  complex_mult_type=use_mults_resources  butterfly_type=use_xtremedsp_slices  simulation_type=hybrid_sim  simulation_model=sysgen:xfftv9_cmodel  data_path_portlist={ 's_axis_data_tdata', 'm_axis_data_tdata', 'm_axis_status_tdata', 'event_fft_overflow' }  channels=1  input_ordering=natural_order  input_width=16  ip_name=Fast Fourier Transform  ip_version=9.0  dsptool_ready=true  ipcore_usecache=true  ipcore_useipmodelcache=true  wrapper_available=true  port_translation_map={ 'aclken' => 'en', 'aresetn' => 'rst'}  data_format=fixed_point  block_type=xfft_v9_0
  Inverter : xbsIndex_r4/Inverter  en=off  latency=0  dbl_ovrd=off  block_type=inv
  Subsystem : Subsystem
  Subsystem1 : Subsystem
  Terminator{3..8} (6 alike) : Terminator
  ready_in : Outport
  valid_out : Outport  Port=2
  data_out : Outport  Port=3
  last_out : Outport  Port=4
  reset_out : Outport  Port=5
  wires:
  data_in/1 -> Subsystem/1(In1)
  IFFT - Fast Fourier Transform 8.1/10 -> Terminator6/1
  IFFT - Fast Fourier Transform 8.1/11 -> Terminator7/1
  IFFT - Fast Fourier Transform 8.1/8 -> Terminator4/1
  IFFT - Fast Fourier Transform 8.1/9 -> Terminator5/1
  IFFT - Fast Fourier Transform 8.1/7 -> Terminator3/1
  Subsystem/1(imag) -> IFFT - Fast Fourier Transform 8.1/3
  IFFT - Fast Fourier Transform 8.1/12 -> Terminator8/1
  Subsystem/2(real) -> IFFT - Fast Fourier Transform 8.1/4
  IFFT/1 -> IFFT - Fast Fourier Transform 8.1/1
  Subsystem1/1(Out1) -> data_out/1
  IFFT - Fast Fourier Transform 8.1/3 -> Subsystem1/1(imag)
  IFFT - Fast Fourier Transform 8.1/1 -> IFFT - Fast Fourier Transform 8.1/2
  IFFT - Fast Fourier Transform 8.1/4 -> Subsystem1/2(real)
  reset_in/1 -> Inverter/1, reset_out/1
  IFFT - Fast Fourier Transform 8.1/6 -> last_out/1
  ready_out/1 -> IFFT - Fast Fourier Transform 8.1/7
  IFFT - Fast Fourier Transform 8.1/5 -> valid_out/1
  valid_in/1 -> IFFT - Fast Fourier Transform 8.1/5
  IFFT - Fast Fourier Transform 8.1/2 -> ready_in/1
  last_in/1 -> IFFT - Fast Fourier Transform 8.1/6
  Inverter/1 -> IFFT - Fast Fourier Transform 8.1/8

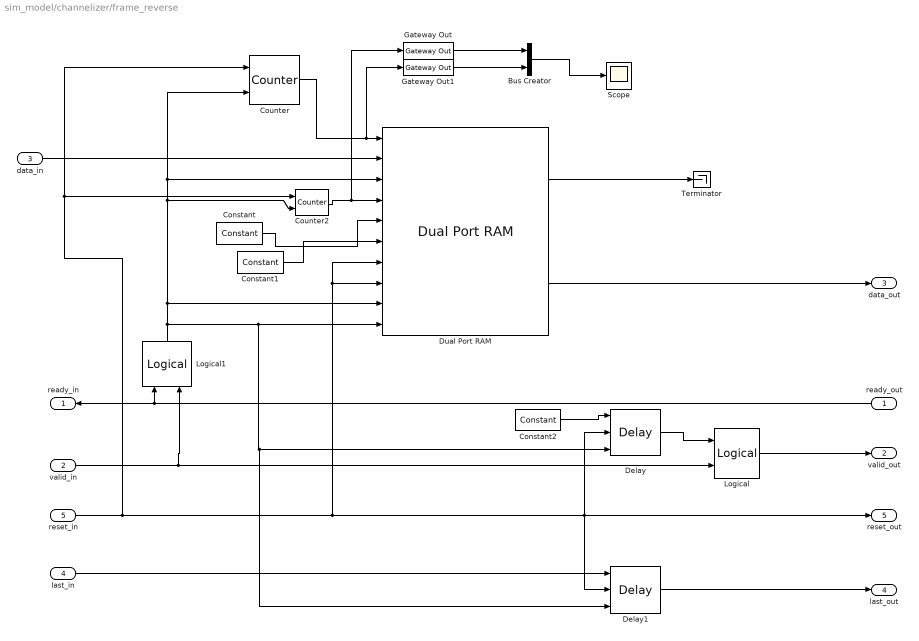
== system sim_model/channelizer/frame_reverse ==
  ready_out : Inport
  valid_in : Inport  Port=2
  data_in : Inport  Port=3
  last_in : Inport  Port=4
  reset_in : Inport  Port=5
  Bus Creator : BusCreator  Inputs=2
  Constant : xbsIndex_r4/Constant  const=0  gui_display_data_type=Fixed-point  arith_type=Unsigned  n_bits=32  bin_pt=0  preci_type=Single  exp_width=8  frac_width=24  explicit_period=off  period=1  equ=P=C  opselect=C  inp2=PCIN>>17  opr=+  inp1=P  carry=CIN  dbl_ovrd=off  block_type=constant
  Constant1 : xbsIndex_r4/Constant  const=0  gui_display_data_type=Boolean  arith_type=Boolean  n_bits=32  bin_pt=0  preci_type=Single  exp_width=8  frac_width=24  explicit_period=off  period=1  equ=P=C  opselect=C  inp2=PCIN>>17  opr=+  inp1=P  carry=CIN  dbl_ovrd=off  block_type=constant
  Constant2 : xbsIndex_r4/Constant  const=1  gui_display_data_type=Boolean  arith_type=Boolean  n_bits=32  bin_pt=0  preci_type=Single  exp_width=8  frac_width=24  explicit_period=off  period=1  equ=P=C  opselect=C  inp2=PCIN>>17  opr=+  inp1=P  carry=CIN  dbl_ovrd=off  block_type=constant
  Counter : xbsIndex_r4/Counter  cnt_type=Free Running  cnt_to=Inf  operation=Up  start_count=0  cnt_by_val=1  arith_type=Unsigned  n_bits=nextpow2(N_sub*2)  bin_pt=0  load_pin=off  rst=on  en=on  explicit_period=on  period=1  use_behavioral_HDL=off  implementation=Fabric  dbl_ovrd=off  block_type=counter
  Counter2 : xbsIndex_r4/Counter  cnt_type=Free Running  cnt_to=Inf  operation=Down  start_count=N_sub*2-1  cnt_by_val=1  arith_type=Unsigned  n_bits=nextpow2(N_sub*2)  bin_pt=0  load_pin=off  rst=on  en=on  explicit_period=on  period=1  use_behavioral_HDL=off  implementation=Fabric  dbl_ovrd=off  block_type=counter
  Delay : xbsIndex_r4/Delay  rst=on  infoeditControl=Selection of Reset will increase slice count due to use of real FFs and instead of SRLs  en=on  latency=1+N_sub  reg_retiming=off  dbl_ovrd=off  block_type=delay
  Delay1 : xbsIndex_r4/Delay  rst=on  infoeditControl=Selection of Reset will increase slice count due to use of real FFs and instead of SRLs  en=on  latency=1  reg_retiming=off  dbl_ovrd=off  block_type=delay
  Dual Port RAM : xbsIndex_r4/Dual Port RAM  depth=2*N_sub  initVector=zeros(1,2+N_sub)  distributed_mem=Block RAM  init_a=0  init_b=0  rst_a=on  rst_b=on  en_a=on  en_b=on  latency=1  write_mode_A=No Read On Write  write_mode_B=No Read On Write  optimize=Area  dbl_ovrd=off  block_type=dpram
  Gateway Out : xbsIndex_r4/Gateway Out  inherit_from_input=off  hdl_port=off  rows=1  columns=1  UseAsDAC=off  DACChannel='1'  interface=None  automatic_assignment=on  address_offset=hex2dec('00')  intf_name=''  intf_description=''  timing_constraint=None  locs_specified=off  LOCs={}  io_standard={}  block_type=gatewayout
  Gateway Out1 : xbsIndex_r4/Gateway Out  inherit_from_input=off  hdl_port=off  rows=1  columns=1  UseAsDAC=off  DACChannel='1'  interface=None  automatic_assignment=on  address_offset=hex2dec('00')  intf_name=''  intf_description=''  timing_constraint=None  locs_specified=off  LOCs={}  io_standard={}  block_type=gatewayout
  Logical : xbsIndex_r4/Logical  logical_function=AND  inputs=2  en=off  latency=0  precision=Full  arith_type=Unsigned  n_bits=16  bin_pt=0  align_bp=on  dbl_ovrd=off  block_type=logical
  Logical1 : xbsIndex_r4/Logical  logical_function=AND  inputs=2  en=off  latency=0  precision=Full  arith_type=Unsigned  n_bits=16  bin_pt=0  align_bp=on  dbl_ovrd=off  block_type=logical
  Scope : Scope
  Terminator : Terminator
  ready_in : Outport
  valid_out : Outport  Port=2
  data_out : Outport  Port=3
  last_out : Outport  Port=4
  reset_out : Outport  Port=5
  wires:
  Constant/1 -> Dual Port RAM/5
  Counter/1 -> Gateway Out1/1, Dual Port RAM/1
  valid_in/1 -> Logical1/2, Logical/2
  ready_out/1 -> Logical1/1, ready_in/1
  Logical1/1 -> Delay1/3, Delay/3, Dual Port RAM/10, Dual Port RAM/9, Counter2/2, Counter/2, Dual Port RAM/3
  Constant1/1 -> Dual Port RAM/6
  reset_in/1 -> Counter2/1, Counter/1, Dual Port RAM/7, Dual Port RAM/8, Delay/2, reset_out/1, Delay1/2
  Counter2/1 -> Gateway Out/1, Dual Port RAM/4
  Dual Port RAM/2 -> data_out/1
  Logical/1 -> valid_out/1
  Delay/1 -> Logical/1
  Dual Port RAM/1 -> Terminator/1
  Bus Creator/1 -> Scope/1
  Gateway Out/1 -> Bus Creator/1
  Gateway Out1/1 -> Bus Creator/2
  Constant2/1 -> Delay/1
  data_in/1 -> Dual Port RAM/2
  Delay1/1 -> last_out/1
  last_in/1 -> Delay1/1

== system sim_model/channelizer/last_handler ==
  ready_out : Inport
  valid_in : Inport  Port=2
  data_in : Inport  Port=3
  last_in : Inport  Port=4
  reset_in : Inport  Port=5
  Constant : xbsIndex_r4/Constant  const=1023  gui_display_data_type=Fixed-point  arith_type=Unsigned  n_bits=nextpow2(1024)  bin_pt=0  preci_type=Single  exp_width=8  frac_width=24  explicit_period=off  period=1  equ=P=C  opselect=C  inp2=PCIN>>17  opr=+  inp1=P  carry=CIN  dbl_ovrd=off  block_type=constant
  Counter : xbsIndex_r4/Counter  cnt_type=Free Running  cnt_to=Inf  operation=Up  start_count=0  cnt_by_val=1  arith_type=Unsigned  n_bits=nextpow2(1024)  bin_pt=0  load_pin=off  rst=on  en=on  explicit_period=on  period=1  use_behavioral_HDL=off  implementation=Fabric  dbl_ovrd=off  block_type=counter
  Logical : xbsIndex_r4/Logical  logical_function=AND  inputs=2  en=off  latency=0  precision=Full  arith_type=Unsigned  n_bits=16  bin_pt=0  align_bp=on  dbl_ovrd=off  block_type=logical
  Relational : xbsIndex_r4/Relational  mode=a=b  op_type=Bool  en=off  latency=0  dbl_ovrd=off  block_type=relational
  Terminator : Terminator
  ready_in : Outport
  valid_out : Outport  Port=2
  data_out : Outport  Port=3
  last_out : Outport  Port=4
  reset_out : Outport  Port=5
  wires:
  reset_in/1 -> Counter/1, reset_out/1
  ready_out/1 -> Logical/2, ready_in/1
  data_in/1 -> data_out/1
  valid_in/1 -> Logical/1, valid_out/1
  last_in/1 -> Terminator/1
  Logical/1 -> Counter/2
  Counter/1 -> Relational/2
  Constant/1 -> Relational/1
  Relational/1 -> last_out/1

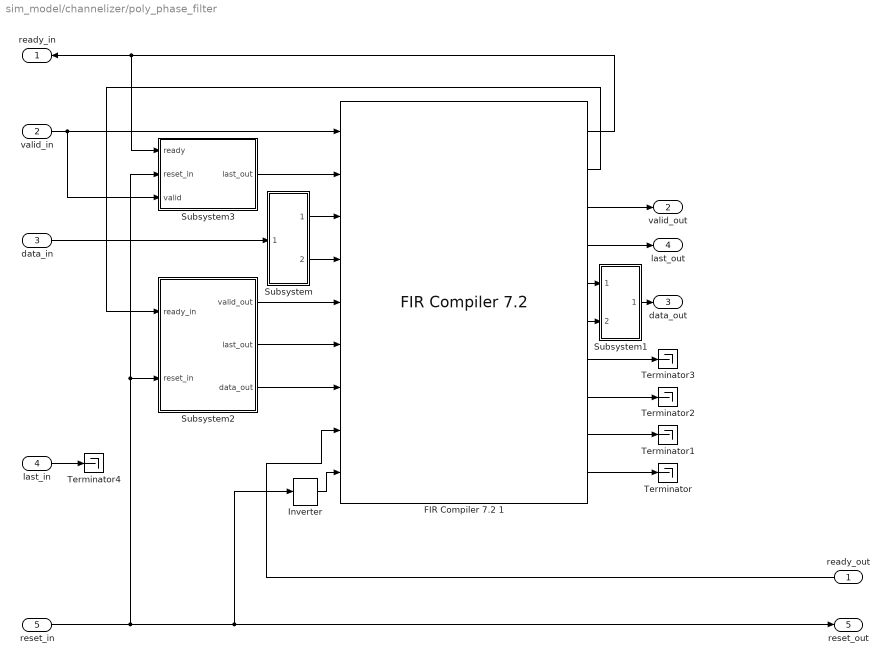
== system sim_model/channelizer/poly_phase_filter ==
  ready_out : Inport
  valid_in : Inport  Port=2
  data_in : Inport  Port=3
  last_in : Inport  Port=4
  reset_in : Inport  Port=5
  FIR Compiler 7.2 1 : xbsIndex_r4/FIR Compiler 7.2   coefficientvector=filt  coefficient_sets=N_sub  coefficient_reload=off  filter_type=Single_Rate  rate_change_type=Integer  interpolation_rate=1  decimation_rate=1  zero_pack_factor=1  channel_sequence=Basic  number_channels=N_sub  pattern_list='P4-0,P4-1,P4-2,P4-3,P4-4'  number_paths=2  ratespecification=Input_Sample_Period  sampleperiod=1  hardwareoversamplingrate=1  coefficient_sign=Signed  quantization=Quantize_Only  coefficient_width=16  bestprecision=off  coefficient_fractional_bits=14  coefficient_structure=Inferred  output_rounding_mode=Full_Precision  output_width=32  filter_architecture=Systolic_Multiply_Accumulate  optimization_goal=Area  optimization_list='None'  data_buffer_type=Automatic  coefficient_buffer_type=Automatic  input_buffer_type=Automatic  output_buffer_type=Automatic  preference_for_other_storage=Automatic  multi_column_support=Automatic  columnconfig='89'  inter_column_pipe_length=4  data_has_tlast=Vector_Framing  m_data_has_tready=on  s_data_has_fifo=on  s_data_has_tuser=Not_Required  m_data_has_tuser=Not_Required  s_config_sync_mode=On_Vector  s_config_method=By_Channel  num_reload_slots=1  has_aclken=off  has_aresetn=on  infoeditControl=ARESETn must be asserted for a minimum of 2 cycles  reset_data_vector=on  trim_axipin_name=on  simulation_type=hybrid_sim  simulation_model=sysgen:xfirv7_2_cmodel  data_path_portlist={ 's_axis_data_tdata', 'm_axis_data_tdata' }  passband_min=0.0  passband_max=0.5  stopband_min=0.5  stopband_max=1.0  filter_selection=1  gui_behaviour='Sysgen_GUI'  data_sign=Signed  data_width=16  data_fractional_bits=0  data_tuser_width=1  wrapper_available=true  ip_wrap_arbitrary_binary_point=true  ip_name=FIR Compiler  ip_version=7.2  dsptool_ready=true  ipcore_usecache=true  ipcore_useipmodelcache=true  port_translation_map={ 'aclken' => 'en', 'aresetn' => 'rst' }  run_core_at_system_period=true  ipcore_xco_need_fpga_part=true  block_type=fir_compiler_v7_2
      settings: infoedit=Maximum Possible : Maximizes oversampling rate. Abstracted input handshake (no s_data_tvalid) and automatic rate propagation.<br>Hardware Oversampling Rate : Specifies oversampling rate relative to the input sample period. Abstracted input handshake (no s_data_tvalid) and automatic rate propagation.<br>Input/Output Sample Period : Specifies absolute oversampling rate. No input handshake abstraction (exposes s_data_tvalid) and no rate propagation.
  Inverter : xbsIndex_r4/Inverter  en=off  latency=0  dbl_ovrd=off  block_type=inv
  Subsystem : Subsystem
  Subsystem1 : Subsystem
  Subsystem2 : Subsystem
  Subsystem3 : Subsystem
  Terminator{,1..4} (5 alike) : Terminator
  ready_in : Outport
  valid_out : Outport  Port=2
  data_out : Outport  Port=3
  last_out : Outport  Port=4
  reset_out : Outport  Port=5
  wires:
  Subsystem1/1(Out1) -> data_out/1
  data_in/1 -> Subsystem/1(In1)
  valid_in/1 -> Subsystem3/3(valid), FIR Compiler 7.2 1/1
  FIR Compiler 7.2 1/1 -> Subsystem3/1(ready), ready_in/1
  FIR Compiler 7.2 1/5 -> Subsystem1/1(imag)
  FIR Compiler 7.2 1/6 -> Subsystem1/2(real)
  ready_out/1 -> FIR Compiler 7.2 1/8
  reset_in/1 -> Inverter/1, reset_out/1, Subsystem2/2(reset_in), Subsystem3/2(reset_in)
  Subsystem/1(imag) -> FIR Compiler 7.2 1/3
  Subsystem/2(real) -> FIR Compiler 7.2 1/4
  Inverter/1 -> FIR Compiler 7.2 1/9
  FIR Compiler 7.2 1/10 -> Terminator/1
  FIR Compiler 7.2 1/9 -> Terminator1/1
  FIR Compiler 7.2 1/8 -> Terminator2/1
  FIR Compiler 7.2 1/7 -> Terminator3/1
  FIR Compiler 7.2 1/3 -> valid_out/1
  FIR Compiler 7.2 1/4 -> last_out/1
  FIR Compiler 7.2 1/2 -> Subsystem2/1(ready_in)
  Subsystem2/3(data_out) -> FIR Compiler 7.2 1/7
  Subsystem2/2(last_out) -> FIR Compiler 7.2 1/6
  Subsystem2/1(valid_out) -> FIR Compiler 7.2 1/5
  Subsystem3/1(last_out) -> FIR Compiler 7.2 1/2
  last_in/1 -> Terminator4/1

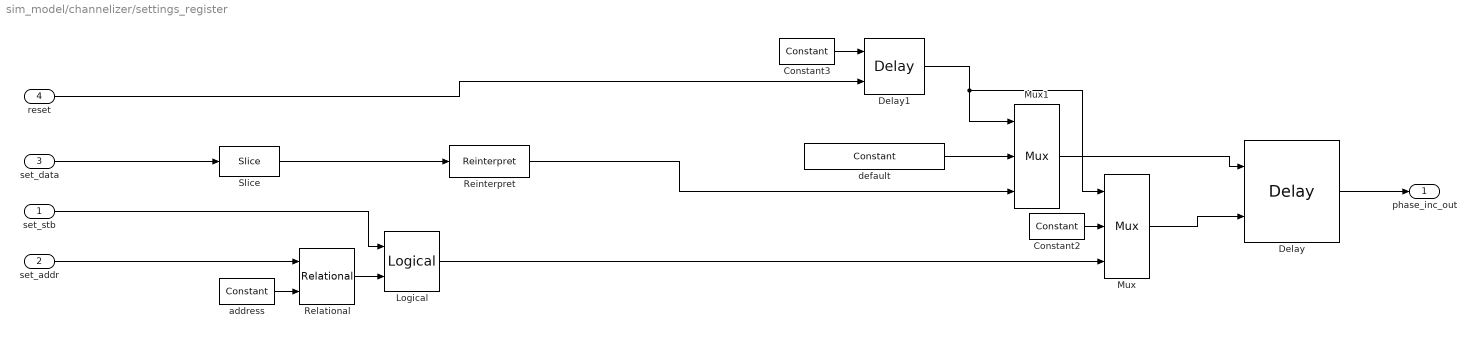
== system sim_model/channelizer/settings_register ==
  set_stb : Inport
  set_addr : Inport  Port=2
  set_data : Inport  Port=3
  reset : Inport  Port=4
  Constant2 : xbsIndex_r4/Constant  const=1.0  gui_display_data_type=Boolean  arith_type=Boolean  n_bits=16  bin_pt=14  preci_type=Single  exp_width=8  frac_width=24  explicit_period=off  period=1  equ=P=C  opselect=C  inp2=PCIN>>17  opr=+  inp1=P  carry=CIN  dbl_ovrd=off  block_type=constant
  Constant3 : xbsIndex_r4/Constant  const=1  gui_display_data_type=Boolean  arith_type=Boolean  n_bits=16  bin_pt=14  preci_type=Single  exp_width=8  frac_width=24  explicit_period=off  period=1  equ=P=C  opselect=C  inp2=PCIN>>17  opr=+  inp1=P  carry=CIN  dbl_ovrd=off  block_type=constant
  Delay : xbsIndex_r4/Delay  rst=off  infoeditControl=Selection of Reset will increase slice count due to use of real FFs and instead of SRLs  en=on  latency=1  reg_retiming=off  dbl_ovrd=off  block_type=delay
  Delay1 : xbsIndex_r4/Delay  rst=on  infoeditControl=Selection of Reset will increase slice count due to use of real FFs and instead of SRLs  en=off  latency=1  reg_retiming=off  dbl_ovrd=off  block_type=delay
  Logical : xbsIndex_r4/Logical  logical_function=AND  inputs=2  en=off  latency=0  precision=Full  arith_type=Unsigned  n_bits=16  bin_pt=0  align_bp=on  dbl_ovrd=off  block_type=logical
  Mux : xbsIndex_r4/Mux  inputs=2  en=off  latency=0  precision=Full  arith_type=Unsigned  n_bits=16  bin_pt=14  quantization=Truncate  overflow=Wrap  dbl_ovrd=off  block_type=mux
  Mux1 : xbsIndex_r4/Mux  inputs=2  en=off  latency=0  precision=Full  arith_type=Unsigned  n_bits=16  bin_pt=14  quantization=Truncate  overflow=Wrap  dbl_ovrd=off  block_type=mux
  Reinterpret : xbsIndex_r4/Reinterpret  force_arith_type=on  arith_type="Signed  (2's comp)"  force_bin_pt=on  bin_pt=modulator_reg_1_num_frac_bits  block_type=reinterpret
  Relational : xbsIndex_r4/Relational  mode=a=b  op_type=Bool  en=off  latency=0  dbl_ovrd=off  block_type=relational
  Slice : xbsIndex_r4/Slice  nbits=1  boolean_output=off  mode=Two Bit Locations  bit1=modulator_reg_1_num_bits-1  base1=LSB of Input  bit0=0  base0=LSB of Input  dbl_ovrd=off  block_type=slice
  address : xbsIndex_r4/Constant  const=modulator_reg_1_address  gui_display_data_type=Fixed-point  arith_type=Unsigned  n_bits=8  bin_pt=0  preci_type=Single  exp_width=8  frac_width=24  explicit_period=off  period=1  equ=P=C  opselect=C  inp2=PCIN>>17  opr=+  inp1=P  carry=CIN  dbl_ovrd=off  block_type=constant
  default : xbsIndex_r4/Constant  const=modulator_reg_1_default  gui_display_data_type=Fixed-point  arith_type=Signed (2's comp)  n_bits=modulator_reg_1_num_bits  bin_pt=modulator_reg_1_num_frac_bits  preci_type=Single  exp_width=8  frac_width=24  explicit_period=off  period=1  equ=P=C  opselect=C  inp2=PCIN>>17  opr=+  inp1=P  carry=CIN  dbl_ovrd=off  block_type=constant
  phase_inc_out : Outport
  wires:
  Relational/1 -> Logical/2
  address/1 -> Relational/2
  Delay/1 -> phase_inc_out/1
  set_data/1 -> Slice/1
  set_stb/1 -> Logical/1
  set_addr/1 -> Relational/1
  Slice/1 -> Reinterpret/1
  Constant3/1 -> Delay1/1
  Delay1/1 -> Mux/1, Mux1/1
  Mux/1 -> Delay/2
  Mux1/1 -> Delay/1
  Constant2/1 -> Mux/2
  default/1 -> Mux1/2
  Logical/1 -> Mux/3
  Reinterpret/1 -> Mux1/3
  reset/1 -> Delay1/2

== system sim_model/channelizer/debug_interface1/Subsystem ==
  In1 : Inport
  Reinterpret : xbsIndex_r4/Reinterpret  force_arith_type=on  arith_type="Signed  (2's comp)"  force_bin_pt=on  bin_pt=15  block_type=reinterpret
  Reinterpret3 : xbsIndex_r4/Reinterpret  force_arith_type=on  arith_type="Signed  (2's comp)"  force_bin_pt=on  bin_pt=15  block_type=reinterpret
  lower : xbsIndex_r4/Slice  nbits=1  boolean_output=off  mode=Two Bit Locations  bit1=15  base1=LSB of Input  bit0=0  base0=LSB of Input  dbl_ovrd=off  block_type=slice
  upper : xbsIndex_r4/Slice  nbits=1  boolean_output=off  mode=Two Bit Locations  bit1=31  base1=LSB of Input  bit0=16  base0=LSB of Input  dbl_ovrd=off  block_type=slice
  Out1 : Outport
  Out2 : Outport  Port=2
  wires:
  lower/1 -> Reinterpret/1
  In1/1 -> lower/1, upper/1
  upper/1 -> Reinterpret3/1
  Reinterpret3/1 -> Out1/1
  Reinterpret/1 -> Out2/1

== system sim_model/channelizer/debug_interface2/Subsystem ==
  In1 : Inport
  Reinterpret : xbsIndex_r4/Reinterpret  force_arith_type=on  arith_type="Signed  (2's comp)"  force_bin_pt=on  bin_pt=15  block_type=reinterpret
  Reinterpret3 : xbsIndex_r4/Reinterpret  force_arith_type=on  arith_type="Signed  (2's comp)"  force_bin_pt=on  bin_pt=15  block_type=reinterpret
  lower : xbsIndex_r4/Slice  nbits=1  boolean_output=off  mode=Two Bit Locations  bit1=15  base1=LSB of Input  bit0=0  base0=LSB of Input  dbl_ovrd=off  block_type=slice
  upper : xbsIndex_r4/Slice  nbits=1  boolean_output=off  mode=Two Bit Locations  bit1=31  base1=LSB of Input  bit0=16  base0=LSB of Input  dbl_ovrd=off  block_type=slice
  Out1 : Outport
  Out2 : Outport  Port=2
  wires:
  lower/1 -> Reinterpret/1
  In1/1 -> lower/1, upper/1
  upper/1 -> Reinterpret3/1
  Reinterpret3/1 -> Out1/1
  Reinterpret/1 -> Out2/1

== system sim_model/channelizer/debug_interface3/Subsystem ==
  In1 : Inport
  Reinterpret : xbsIndex_r4/Reinterpret  force_arith_type=on  arith_type="Signed  (2's comp)"  force_bin_pt=on  bin_pt=15  block_type=reinterpret
  Reinterpret3 : xbsIndex_r4/Reinterpret  force_arith_type=on  arith_type="Signed  (2's comp)"  force_bin_pt=on  bin_pt=15  block_type=reinterpret
  lower : xbsIndex_r4/Slice  nbits=1  boolean_output=off  mode=Two Bit Locations  bit1=15  base1=LSB of Input  bit0=0  base0=LSB of Input  dbl_ovrd=off  block_type=slice
  upper : xbsIndex_r4/Slice  nbits=1  boolean_output=off  mode=Two Bit Locations  bit1=31  base1=LSB of Input  bit0=16  base0=LSB of Input  dbl_ovrd=off  block_type=slice
  Out1 : Outport
  Out2 : Outport  Port=2
  wires:
  Reinterpret/1 -> Out2/1
  Reinterpret3/1 -> Out1/1
  upper/1 -> Reinterpret3/1
  In1/1 -> upper/1, lower/1
  lower/1 -> Reinterpret/1

== system sim_model/channelizer/debug_interface4/Subsystem ==
  In1 : Inport
  Reinterpret : xbsIndex_r4/Reinterpret  force_arith_type=on  arith_type="Signed  (2's comp)"  force_bin_pt=on  bin_pt=15  block_type=reinterpret
  Reinterpret3 : xbsIndex_r4/Reinterpret  force_arith_type=on  arith_type="Signed  (2's comp)"  force_bin_pt=on  bin_pt=15  block_type=reinterpret
  lower : xbsIndex_r4/Slice  nbits=1  boolean_output=off  mode=Two Bit Locations  bit1=15  base1=LSB of Input  bit0=0  base0=LSB of Input  dbl_ovrd=off  block_type=slice
  upper : xbsIndex_r4/Slice  nbits=1  boolean_output=off  mode=Two Bit Locations  bit1=31  base1=LSB of Input  bit0=16  base0=LSB of Input  dbl_ovrd=off  block_type=slice
  Out1 : Outport
  Out2 : Outport  Port=2
  wires:
  lower/1 -> Reinterpret/1
  In1/1 -> lower/1, upper/1
  upper/1 -> Reinterpret3/1
  Reinterpret3/1 -> Out1/1
  Reinterpret/1 -> Out2/1

== system sim_model/channelizer/debug_interface5/Subsystem ==
  In1 : Inport
  Reinterpret : xbsIndex_r4/Reinterpret  force_arith_type=on  arith_type="Signed  (2's comp)"  force_bin_pt=on  bin_pt=15  block_type=reinterpret
  Reinterpret3 : xbsIndex_r4/Reinterpret  force_arith_type=on  arith_type="Signed  (2's comp)"  force_bin_pt=on  bin_pt=15  block_type=reinterpret
  lower : xbsIndex_r4/Slice  nbits=1  boolean_output=off  mode=Two Bit Locations  bit1=15  base1=LSB of Input  bit0=0  base0=LSB of Input  dbl_ovrd=off  block_type=slice
  upper : xbsIndex_r4/Slice  nbits=1  boolean_output=off  mode=Two Bit Locations  bit1=31  base1=LSB of Input  bit0=16  base0=LSB of Input  dbl_ovrd=off  block_type=slice
  Out1 : Outport
  Out2 : Outport  Port=2
  wires:
  lower/1 -> Reinterpret/1
  In1/1 -> lower/1, upper/1
  upper/1 -> Reinterpret3/1
  Reinterpret3/1 -> Out1/1
  Reinterpret/1 -> Out2/1

== system sim_model/channelizer/fft1/Subsystem ==
  In1 : Inport
  Reinterpret : xbsIndex_r4/Reinterpret  force_arith_type=on  arith_type="Signed  (2's comp)"  force_bin_pt=on  bin_pt=15  block_type=reinterpret
  Reinterpret1 : xbsIndex_r4/Reinterpret  force_arith_type=on  arith_type="Signed  (2's comp)"  force_bin_pt=on  bin_pt=15  block_type=reinterpret
  Slice : xbsIndex_r4/Slice  nbits=1  boolean_output=off  mode=Two Bit Locations  bit1=15  base1=LSB of Input  bit0=0  base0=LSB of Input  dbl_ovrd=off  block_type=slice
  Slice1 : xbsIndex_r4/Slice  nbits=1  boolean_output=off  mode=Two Bit Locations  bit1=31  base1=LSB of Input  bit0=16  base0=LSB of Input  dbl_ovrd=off  block_type=slice
  imag : Outport
  real : Outport  Port=2
  wires:
  Reinterpret1/1 -> imag/1
  In1/1 -> Slice1/1, Slice/1
  Reinterpret/1 -> real/1
  Slice1/1 -> Reinterpret1/1
  Slice/1 -> Reinterpret/1

== system sim_model/channelizer/fft1/Subsystem1 ==
  imag : Inport
  real : Inport  Port=2
  Concat : xbsIndex_r4/Concat  num_inputs=2  dbl_ovrd=off  block_type=concat
  Convert : xbsIndex_r4/Convert  gui_display_data_type=Fixed-point  arith_type="Signed  (2's comp)"  n_bits=16  bin_pt=13  float_type=Single  exp_bits=8  fraction_bits=24  quantization=Truncate  overflow=Saturate  en=off  latency=0  pipeline=off  dbl_ovrd=off  block_type=convert
  Convert2 : xbsIndex_r4/Convert  gui_display_data_type=Fixed-point  arith_type="Signed  (2's comp)"  n_bits=16  bin_pt=13  float_type=Single  exp_bits=8  fraction_bits=24  quantization=Truncate  overflow=Saturate  en=off  latency=0  pipeline=off  dbl_ovrd=off  block_type=convert
  Reinterpret1 : xbsIndex_r4/Reinterpret  force_arith_type=on  arith_type=Unsigned  force_bin_pt=on  bin_pt=0  block_type=reinterpret
  Reinterpret2 : xbsIndex_r4/Reinterpret  force_arith_type=on  arith_type=Unsigned  force_bin_pt=on  bin_pt=0  block_type=reinterpret
  Out1 : Outport
  wires:
  Reinterpret1/1 -> Concat/2
  imag/1 -> Convert/1
  Concat/1 -> Out1/1
  Reinterpret2/1 -> Concat/1
  real/1 -> Convert2/1
  Convert/1 -> Reinterpret2/1
  Convert2/1 -> Reinterpret1/1

== system sim_model/channelizer/poly_phase_filter/Subsystem ==
  In1 : Inport
  Convert : xbsIndex_r4/Convert  gui_display_data_type=Fixed-point  arith_type="Signed  (2's comp)"  n_bits=18  bin_pt=0  float_type=Single  exp_bits=8  fraction_bits=24  quantization=Truncate  overflow=Wrap  en=off  latency=0  pipeline=off  dbl_ovrd=off  block_type=convert
  Convert1 : xbsIndex_r4/Convert  gui_display_data_type=Fixed-point  arith_type="Signed  (2's comp)"  n_bits=18  bin_pt=0  float_type=Single  exp_bits=8  fraction_bits=24  quantization=Truncate  overflow=Wrap  en=off  latency=0  pipeline=off  dbl_ovrd=off  block_type=convert
  Reinterpret : xbsIndex_r4/Reinterpret  force_arith_type=on  arith_type="Signed  (2's comp)"  force_bin_pt=on  bin_pt=0  block_type=reinterpret
  Reinterpret3 : xbsIndex_r4/Reinterpret  force_arith_type=on  arith_type="Signed  (2's comp)"  force_bin_pt=on  bin_pt=0  block_type=reinterpret
  lower : xbsIndex_r4/Slice  nbits=1  boolean_output=off  mode=Two Bit Locations  bit1=15  base1=LSB of Input  bit0=0  base0=LSB of Input  dbl_ovrd=off  block_type=slice
  upper : xbsIndex_r4/Slice  nbits=1  boolean_output=off  mode=Two Bit Locations  bit1=31  base1=LSB of Input  bit0=16  base0=LSB of Input  dbl_ovrd=off  block_type=slice
  imag : Outport
  real : Outport  Port=2
  wires:
  lower/1 -> Reinterpret/1
  Reinterpret/1 -> Convert1/1
  In1/1 -> lower/1, upper/1
  upper/1 -> Reinterpret3/1
  Reinterpret3/1 -> Convert/1
  Convert/1 -> imag/1
  Convert1/1 -> real/1
